simulink model "FiltroKalamananalisis"  (R2015a)
settings: Solver=ode3  StartTime=0.0  StopTime=50  FixedStep=0.01  RelTol=1e-3
undefined symbols (not defined in the file or in its folder): Discrete, Time
libraries: ctrlSharedLib x1
settings Model: Creator=Brayan  LastModifiedBy=Brayan

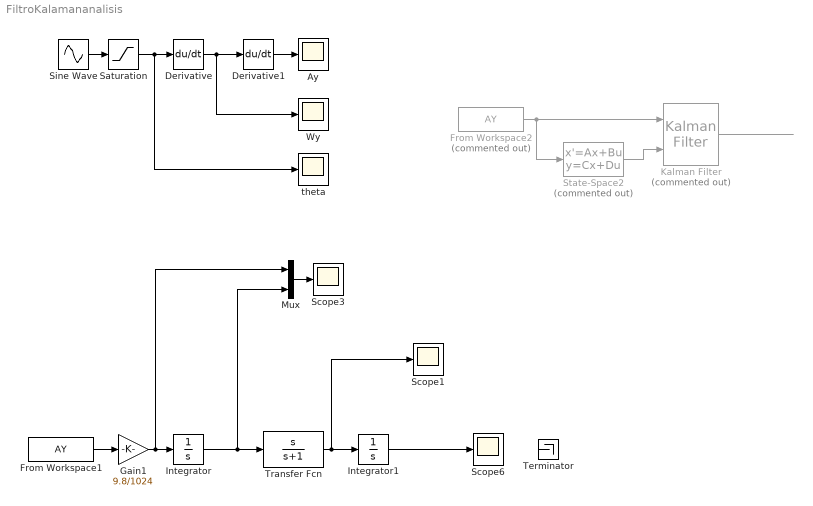
== system FiltroKalamananalisis ==
  Ay : Scope
      settings: SaveName=ScopeData2
  Derivative : Derivative
  Derivative1 : Derivative
  From Workspace1 : FromWorkspace  VariableName=AY  SampleTime=0  OutputAfterFinalValue=Holding final value
  From Workspace2 : FromWorkspace  Commented=on  VariableName=AY  SampleTime=0  OutputAfterFinalValue=Holding final value
  Gain1 : Gain  Gain=9.8/1024
  Integrator : Integrator
  Integrator1 : Integrator
  Kalman Filter : ctrlSharedLib/Kalman Filter  Commented=on  TimeDomain=Discrete-Time  UseCurrentEstimator=on  ModelSource=Individual A, B, C, D matrices  ModelSourceVariable=ss(0.95,1,1,0,1)  A=[0 1; 0 0]  B=[0; 0.60]  C=[1 0]  D=0  NumberOfStates=1  NumberOfInputs=1  NumberOfOutputs=1  InitialEstimateSource=Dialog  X0=0  P0=10  UseK=off  UseGH=off  NumberOfProcessNoiseInputs=1  G=1  TimeInvariantG=on  H=0  TimeInvariantH=on  Q=0.05  TimeInvariantQ=on  R=1  TimeInvariantR=on  N=0  TimeInvariantN=on  AddInputPort=on  AddEnablePort=off  OutputEstimatedY=off  OutputP=off  Ts=-1
  Mux : Mux  Inputs=2
  Saturation : Saturate  UpperLimit=pi/2  LowerLimit=0
  Scope1 : Scope
      settings: SaveName=ScopeData4
  Scope3 : Scope
      settings: SaveName=ScopeData3
  Scope6 : Scope
      settings: SaveName=ScopeData6
  Sine Wave : Sin  Amplitude=pi/2  SampleTime=0
  State-Space2 : StateSpace  Commented=on  A=[0 1; 0 0]  B=[0; 0.60]  C=[1 0]  D=0  X0=0
  Terminator : Terminator
  Transfer Fcn : TransferFcn  Numerator=[1 0]  Denominator=[1 1]
  Wy : Scope
  theta : Scope
  wires:
  Sine Wave/1 -> Saturation/1
  Saturation/1 -> Derivative/1, theta/1
  Derivative/1 -> Derivative1/1, Wy/1
  Derivative1/1 -> Ay/1
  From Workspace1/1 -> Gain1/1
  Gain1/1 -> Mux/1, Integrator/1
  Integrator1/1 -> Scope6/1
  Integrator/1 -> Transfer Fcn/1, Mux/2
  Mux/1 -> Scope3/1
  Kalman Filter/1 -> ?
  From Workspace2/1 -> State-Space2/1, Kalman Filter/1
  State-Space2/1 -> Kalman Filter/2
  Transfer Fcn/1 -> Scope1/1, Integrator1/1
